simulink model "earthquake"  (R2024b)
settings: Solver=FixedStepAuto  StartTime=0.0  StopTime=20  FixedStep=0.001  RelTol=1e-3
values from neighbouring files (symbols this model uses):
  c = 0.5    [GUI.m]    (also in analytical.m = 80; earthquake.m = 100)
  k = 100.0    (= 100)    [GUI.m]    (also in analytical.m = 60000; earthquake.m = 60000)
  m = 1.0    (= 1)    [GUI.m]    (also in analytical.m = 3000; earthquake.m = 4000)
settings Model: Creator=jasad  LastModifiedBy=Fateh

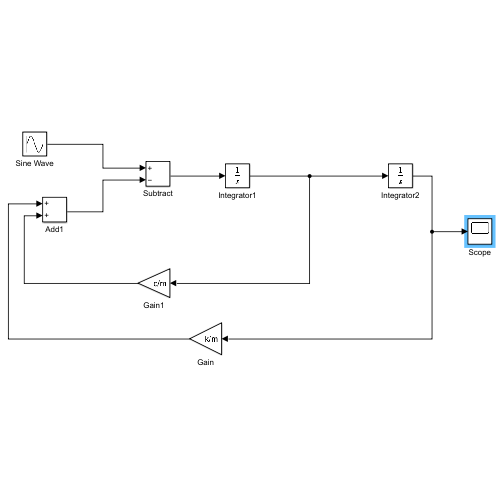
[thumbnail: Simulink's stored preview of the top-level diagram]
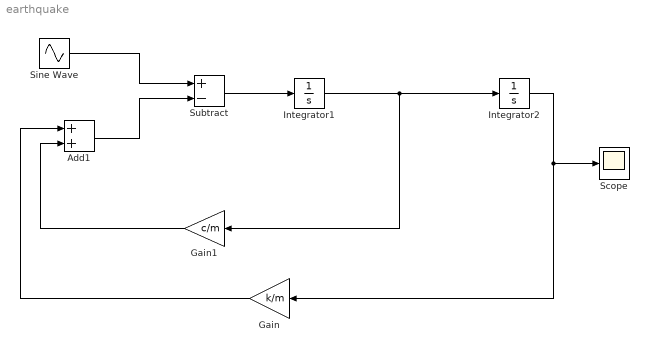
== system earthquake ==
  Add1 : Sum
  Gain : Gain  Gain=k/m
  Gain1 : Gain  Gain=c/m
  Integrator1 : Integrator
  Integrator2 : Integrator
  Scope : Scope
  Sine Wave : Sin  Amplitude=0.2  Frequency=2*pi*1.5  SampleTime=0
  Subtract : Sum  Inputs=+-
  wires:
  Integrator1/1 -> Gain1/1, Integrator2/1
  Integrator2/1 -> Scope/1, Gain/1
  Gain1/1 -> Add1/2
  Gain/1 -> Add1/1
  Sine Wave/1 -> Subtract/1
  Add1/1 -> Subtract/2
  Subtract/1 -> Integrator1/1
